simulink model "NonLinearModelDevelopment_Example"  (R2015a)
settings: Solver=ode45  StartTime=0.0  StopTime=10.0  RelTol=1e-3
InitFcn:
  | Suspension_Parameters_2021
undefined symbols (not defined in the file): bs, bsn, Initial, ks, ksn, kt, magnitude, mb, mw
settings Model: Creator=user  LastModifiedBy=user

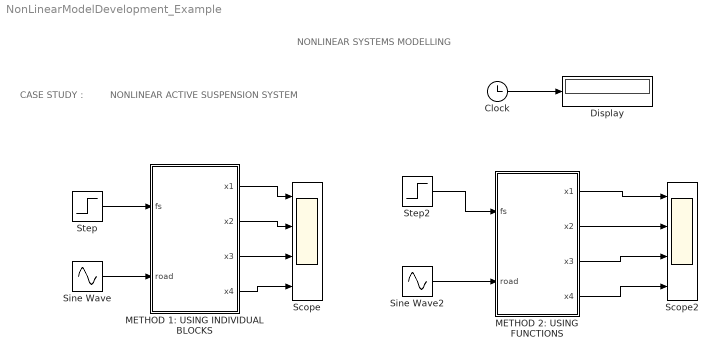
== system NonLinearModelDevelopment_Example ==
  note: NONLINEAR ACTIVE SUSPENSION SYSTEM
  note: CASE STUDY :
  note: NONLINEAR SYSTEMS MODELLING
  Clock : Clock
  Display : Display
  METHOD 1: USING INDIVIDUAL BLOCKS : Subsystem
  METHOD 2: USING FUNCTIONS : Subsystem
  Scope : Scope  NumInputPorts=4
      settings: YMin=-5~-5~-5~-5  YMax=5~5~5~5
  Scope2 : Scope  NumInputPorts=4
      settings: YMin=-5~-5~-5~-5  YMax=5~5~5~5  SaveName=ScopeData2
  Sine Wave : Sin  Amplitude=0.01  SampleTime=0
  Sine Wave2 : Sin  Amplitude=0.01  SampleTime=0
  Step : Step  SampleTime=0
  Step2 : Step  SampleTime=0
  wires:
  METHOD 1: USING INDIVIDUAL BLOCKS/1(x1) -> Scope/1
  METHOD 1: USING INDIVIDUAL BLOCKS/2(x2) -> Scope/2
  METHOD 1: USING INDIVIDUAL BLOCKS/3(x3) -> Scope/3
  METHOD 1: USING INDIVIDUAL BLOCKS/4(x4) -> Scope/4
  Step/1 -> METHOD 1: USING INDIVIDUAL BLOCKS/1(fs)
  Sine Wave/1 -> METHOD 1: USING INDIVIDUAL BLOCKS/2(road)
  Clock/1 -> Display/1
  Step2/1 -> METHOD 2: USING FUNCTIONS/1(fs)
  Sine Wave2/1 -> METHOD 2: USING FUNCTIONS/2(road)
  METHOD 2: USING FUNCTIONS/1(x1) -> Scope2/1
  METHOD 2: USING FUNCTIONS/2(x2) -> Scope2/2
  METHOD 2: USING FUNCTIONS/3(x3) -> Scope2/3
  METHOD 2: USING FUNCTIONS/4(x4) -> Scope2/4

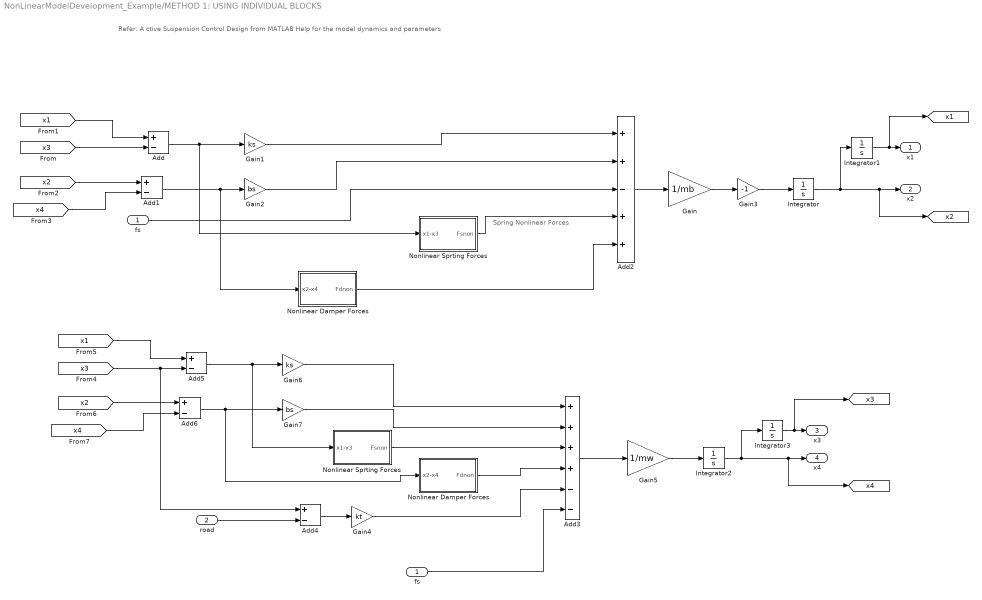
== system NonLinearModelDevelopment_Example/METHOD 1: USING INDIVIDUAL BLOCKS ==
  note: Spring Nonlinear Forces
  note: Refer: A ctive Suspension Control Design from MATLAB Help for the model dynamics and parameters
  fs : Inport
  road : Inport  Port=2
  Add{,1,4..6} (5 alike) : Sum  Inputs=+-
  Add2 : Sum  Inputs=++-++
  Add3 : Sum  Inputs=++++--
  Gain : Gain  Gain=1/mb
  Gain1 : Gain  Gain=ks
  Gain2 : Gain  Gain=bs
  Gain3 : Gain  Gain=-1
  Gain4 : Gain  Gain=kt
  Gain5 : Gain  Gain=1/mw
  Gain6 : Gain  Gain=ks
  Gain7 : Gain  Gain=bs
  Integrator : Integrator  InitialCondition=Initial.x2
  Integrator1 : Integrator  InitialCondition=Initial.x1
  Integrator2 : Integrator  InitialCondition=Initial.x4
  Integrator3 : Integrator  InitialCondition=Initial.x3
  Nonlinear Damper Forces : Subsystem
  "Nonlinear Damper Forces   " : Subsystem
  Nonlinear Sprting Forces : Subsystem
  "Nonlinear Sprting Forces   " : Subsystem
  "fs  " : InportShadow
  x1 : Outport
  x2 : Outport  Port=2
  x3 : Outport  Port=3
  x4 : Outport  Port=4
  tag scope: x1=global, x2=global, x3=global, x4=global
  wires:
  Add/1 -> Nonlinear Sprting Forces/1(x1-x3), Gain1/1
  Add1/1 -> Nonlinear Damper Forces/1(x2-x4), Gain2/1
  Integrator1/1 -> [x1], x1/1
  Integrator3/1 -> [x3], x3/1
  Integrator/1 -> Integrator1/1, [x2], x2/1
  Integrator2/1 -> Integrator3/1, [x4], x4/1
  Gain1/1 -> Add2/1
  Gain2/1 -> Add2/2
  fs/1 -> Add2/3
  Add2/1 -> Gain/1
  Gain/1 -> Gain3/1
  Gain3/1 -> Integrator/1
  road/1 -> Add4/2
  Add4/1 -> Gain4/1
  Add3/1 -> Gain5/1
  Gain5/1 -> Integrator2/1
  Nonlinear Sprting Forces/1(Fsnon) -> Add2/4
  Nonlinear Damper Forces/1(Fdnon) -> Add2/5
  [x3] -> Add/2
  [x1] -> Add/1
  [x2] -> Add1/1
  [x4] -> Add1/2
  "Nonlinear Sprting Forces   "/1(Fsnon) -> Add3/3
  "Nonlinear Damper Forces   "/1(Fdnon) -> Add3/4
  Gain4/1 -> Add3/5
  "fs  "/1 -> Add3/6
  Add5/1 -> "Nonlinear Sprting Forces   "/1(x1-x3), Gain6/1
  Add6/1 -> "Nonlinear Damper Forces   "/1(x2-x4), Gain7/1
  [x3] -> Add4/1, Add5/2
  [x1] -> Add5/1
  [x2] -> Add6/1
  [x4] -> Add6/2
  Gain7/1 -> Add3/2
  Gain6/1 -> Add3/1

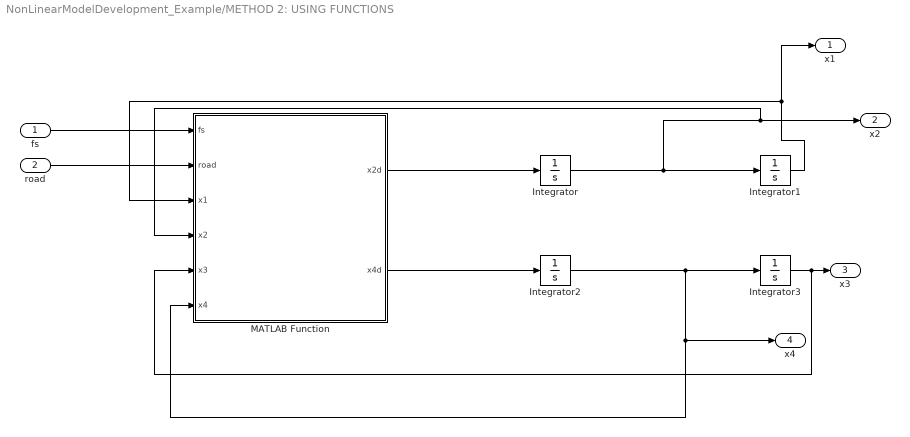
== system NonLinearModelDevelopment_Example/METHOD 2: USING FUNCTIONS ==
  fs : Inport
  road : Inport  Port=2
  Integrator : Integrator  InitialCondition=Initial.x2
  Integrator1 : Integrator  InitialCondition=Initial.x1
  Integrator2 : Integrator  InitialCondition=Initial.x4
  Integrator3 : Integrator  InitialCondition=Initial.x3
  MATLAB Function : MATLAB Function  TreatAsAtomicUnit=on
  x1 : Outport
  x2 : Outport  Port=2
  x3 : Outport  Port=3
  x4 : Outport  Port=4
  wires:
  MATLAB Function/1(x2d) -> Integrator/1
  Integrator/1 -> MATLAB Function/4(x2), x2/1, Integrator1/1
  MATLAB Function/2(x4d) -> Integrator2/1
  Integrator2/1 -> x4/1, MATLAB Function/6(x4), Integrator3/1
  Integrator1/1 -> x1/1, MATLAB Function/3(x1)
  Integrator3/1 -> MATLAB Function/5(x3), x3/1
  road/1 -> MATLAB Function/2(road)
  fs/1 -> MATLAB Function/1(fs)

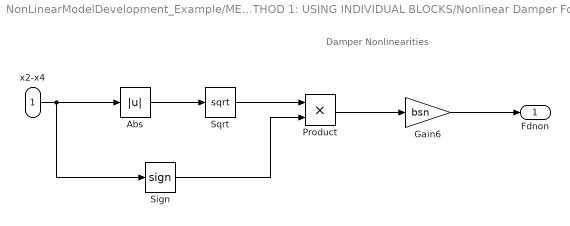
== system NonLinearModelDevelopment_Example/METHOD 1: USING INDIVIDUAL BLOCKS/Nonlinear Damper Forces ==
  note: Damper Nonlinearities
  x2-x4 : Inport
  Abs : Abs
  Gain6 : Gain  Gain=bsn
  Product : Product
  Sign : Signum
  Sqrt : Sqrt  SaturateOnIntegerOverflow=on
  Fdnon : Outport
  wires:
  Product/1 -> Gain6/1
  Gain6/1 -> Fdnon/1
  x2-x4/1 -> Sign/1, Abs/1
  Abs/1 -> Sqrt/1
  Sqrt/1 -> Product/1
  Sign/1 -> Product/2

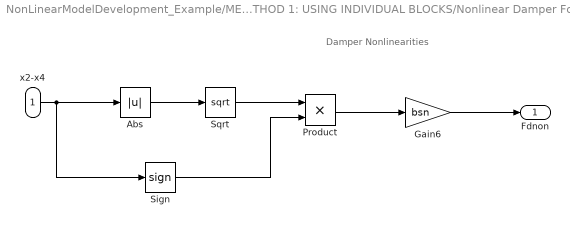
== system NonLinearModelDevelopment_Example/METHOD 1: USING INDIVIDUAL BLOCKS/Nonlinear Damper Forces    ==
  note: Damper Nonlinearities
  x2-x4 : Inport
  Abs : Abs
  Gain6 : Gain  Gain=bsn
  Product : Product
  Sign : Signum
  Sqrt : Sqrt  SaturateOnIntegerOverflow=on
  Fdnon : Outport
  wires:
  Product/1 -> Gain6/1
  Gain6/1 -> Fdnon/1
  x2-x4/1 -> Sign/1, Abs/1
  Abs/1 -> Sqrt/1
  Sqrt/1 -> Product/1
  Sign/1 -> Product/2

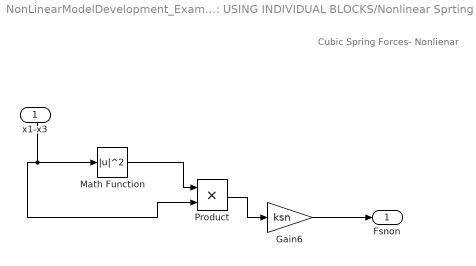
== system NonLinearModelDevelopment_Example/METHOD 1: USING INDIVIDUAL BLOCKS/Nonlinear Sprting Forces ==
  note: Cubic Spring Forces- Nonlienar
  x1-x3 : Inport
  Gain6 : Gain  Gain=ksn
  Math Function : Math  Operator=magnitude^2  SaturateOnIntegerOverflow=on
  Product : Product
  Fsnon : Outport
  wires:
  x1-x3/1 -> Product/2, Math Function/1
  Product/1 -> Gain6/1
  Gain6/1 -> Fsnon/1
  Math Function/1 -> Product/1

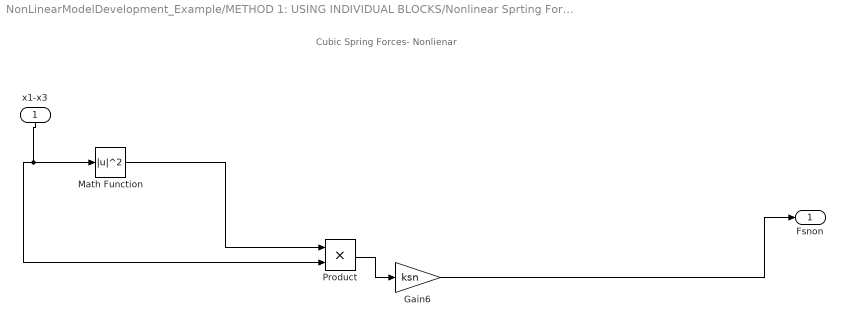
== system NonLinearModelDevelopment_Example/METHOD 1: USING INDIVIDUAL BLOCKS/Nonlinear Sprting Forces    ==
  note: Cubic Spring Forces- Nonlienar
  x1-x3 : Inport
  Gain6 : Gain  Gain=ksn
  Math Function : Math  Operator=magnitude^2  SaturateOnIntegerOverflow=on
  Product : Product
  Fsnon : Outport
  wires:
  x1-x3/1 -> Product/2, Math Function/1
  Product/1 -> Gain6/1
  Gain6/1 -> Fsnon/1
  Math Function/1 -> Product/1

== matlab function NonLinearModelDevelopment_Example/METHOD 2: USING FUNCTIONS/MATLAB Function ==
  data: fs input; x2d output; road input; x4d output; x1 input; x2 input; x3 input; x4 input
function [x2d,x4d] = fcn(fs,road,x1,x2,x3,x4)
%#codegen

mb = 300;    % kg
mw = 60;     % kg
bs = 1000;   % N/m/s
ks = 16000 ; % N/m
kt = 190000; % N/m
ksn = 0.1*ks; 
bsn = 0.1*bs;


x2d = -(1/mb)*(ks*(x1-x3)+ bs*(x2-x4)- fs + ksn*(x1-x3)^3 + bsn*sqrt(abs(x2-x4))*sign(x2-x4));
x4d = (1/mw)*(ks*(x1-x3)+bs*(x2-x4)-kt*(x3-road)-fs + ksn*(x1-x3)^3 + bsn*sqrt(abs(x2-x4))*sign(x2-x4));
